simulink model "simplemedusa_model"  (R2020a)
settings: Solver=VariableStepAuto  StartTime=0.0  StopTime=CONSTANTS.T  RelTol=1e-3
model workspace (MAT data in the model file):
  CONSTANTS.MODELPARAMS.mass = 17
  CONSTANTS.MODELPARAMS.I_z = 1
  CONSTANTS.MODELPARAMS.X_dot_u = -20
  CONSTANTS.MODELPARAMS.Y_dot_v = -30
  CONSTANTS.MODELPARAMS.N_dot_r = -8.69
  CONSTANTS.MODELPARAMS.X_u = -0.2
  CONSTANTS.MODELPARAMS.Y_v = -50
  CONSTANTS.MODELPARAMS.N_r = -4.14
  CONSTANTS.MODELPARAMS.X_uu = -25
  CONSTANTS.MODELPARAMS.Y_vv = -0.01
  CONSTANTS.MODELPARAMS.N_rr = -6.23
  CONSTANTS.MODELPARAMS.m_u = 37
  CONSTANTS.MODELPARAMS.m_v = 47
  CONSTANTS.MODELPARAMS.m_r = 9.69
  CONSTANTS.MODELPARAMS.m_uv = -10
  CONSTANTS.MODELPARAMS.fu = 0
  CONSTANTS.MODELPARAMS.fv = 0
  CONSTANTS.MODELPARAMS.fr = 0
  CONSTANTS.MODELPARAMS.Vcx = 0
  CONSTANTS.MODELPARAMS.Vcy = 0
  CONSTANTS.T = 15
  CONSTANTS.xi = [0 0 0 1 0 0]
  CONSTANTS.xf = [15 0 0 1 0 0]
  CONSTANTS.N = 30
  CONSTANTS.obstacles = []
  CONSTANTS.obstacles_circles = []
  CONSTANTS.min_dist_intervehicles = 3
  CONSTANTS.DiffMat = [-2 -0.0666666666667 0 0 0 0 0 0 0 0 0 0 ... (961 elements, 31x31)]
  CONSTANTS.EvalMat = [1 0.361661513462 0.1262127701 0.0423911582752 0.0136635263144 0.00421272023309 0.00123794003929 0.00034530068424 9.10002914127e-05 2.25393402907e-05 5.21509505085e-06 1.11936155556e-06 ... (961 elements, 31x31)]
  CONSTANTS.BigElevMat = [1 0.9 0.809698996656 0.728185674845 0.654631566274 0.588283772395 0.528458304016 0.47453398728 0.425946889606 0.382185222866 0.342784684426 0.30732419983 ... (9331 elements, 301x31)]
  CONSTANTS.numvars = 6
  CONSTANTS.numinputs = 2
  CONSTANTS.Nv = 1
  CONSTANTS.uselogbar = 0
  CONSTANTS.usesigma = 1
  CONSTANTS.statebounds = [-100  -100  -100  -100  -100  -100; 100  100  100  100  100  100]
  CONSTANTS.inputbounds = [-100  -500; 100  500]
  CONSTANTS.costfun_single : function handle (value not decoded)
  CONSTANTS.dynamics : function handle (value not decoded)
  CONSTANTS.init_guess : function handle (value not decoded)
  CONSTANTS.recoverxy : function handle (value not decoded)
  init_vals = [0 0 0 1 0 0]
  tau_r = [43.137679435; -49.2714696293; 18.7459499295; -4.54662431489; 6.658047137; 13.2270237858; 11.3261149802; -5.40954170829; 2.88065093377; -8.94479642329; -0.278054380158; -1.20355590744; 3.44120490313; 2.32411595817; -0.203876719026; 1.93362993926; -0.957580280562; -0.359407602556; 1.46637180945; -1.70192437834; 1.82794903823; -1.09013224286; 0.795656971372; -0.229115148479; 0.177399034781; -0.0352838490099; -0.0922338252967; -0.23784107908; -0.358640517482; -0.316734931346; 0.333994448023]
  tau_u = [19.7607060301; 12.9276910923; 5.53573475394; 4.05635814498; -0.69958092646; 4.06715022134; -3.35509577272; 4.00552304303; -5.80965699996; 11.9065756877; -1.60028180312; 19.6479288494; 1.90021340601; 15.5960881126; 7.73787556532; 8.16534647911; 12.3908641622; 5.37909869708; 12.5613293191; 6.97515929299; 10.8367698131; 8.90302526194; 10.1461113341; 10.1316611384; 10.871270906; 11.7672320885; 13.2342568079; 15.5312905623; 19.2247320659; 25.3375478214; 35.9280012744]
settings Model: Creator=thomas  LastModifiedBy=thomas

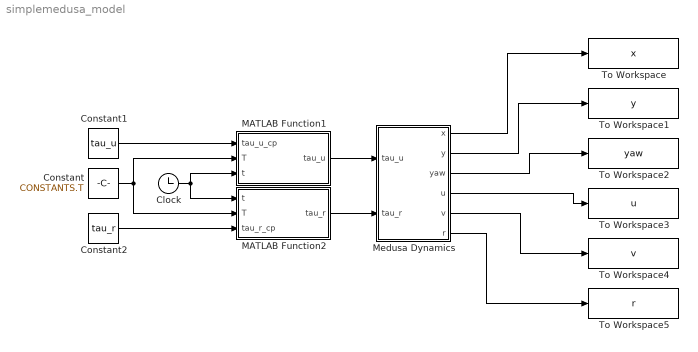
== system simplemedusa_model ==
  Clock : Clock
  Constant : Constant  Value=CONSTANTS.T
  Constant1 : Constant  Value=tau_u
  Constant2 : Constant  Value=tau_r
  MATLAB Function1 : MATLAB Function  TreatAsAtomicUnit=on
  MATLAB Function2 : MATLAB Function  TreatAsAtomicUnit=on
  Medusa Dynamics : Subsystem  mask{x0=init_vals(1), y0=init_vals(2), yaw0=init_vals(3), u0=init_vals(4), v0=init_vals(5), r0=init_vals(6), dist_u=CONSTANTS.MODELPARAMS.fu, dist_v=CONSTANTS.MODELPARAMS.fv, dist_r=CONSTANTS.MODELPARAMS.fr, Vcx=CONSTANTS.MODELPARAMS.Vcx, Vcy=CONSTANTS.MODELPARAMS.Vcy}
      mask prompts: dist_u "Disturbance in u"; dist_v "Disturbance in v"; dist_r "Disturbance in r"; Vcx "Current x"; Vcy "Current y"
  To Workspace : ToWorkspace  VariableName=x  SaveFormat=Structure With Time  SampleTime=-1
  To Workspace1 : ToWorkspace  VariableName=y  SaveFormat=Structure With Time  SampleTime=-1
  To Workspace2 : ToWorkspace  VariableName=yaw  SaveFormat=Structure With Time  SampleTime=-1
  To Workspace3 : ToWorkspace  VariableName=u  SaveFormat=Structure With Time  SampleTime=-1
  To Workspace4 : ToWorkspace  VariableName=v  SaveFormat=Structure With Time  SampleTime=-1
  To Workspace5 : ToWorkspace  VariableName=r  SaveFormat=Structure With Time  SampleTime=-1
  wires:
  MATLAB Function1/1(tau_u) -> Medusa Dynamics/1(tau_u)
  Clock/1 -> MATLAB Function2/1(t), MATLAB Function1/3(t)
  MATLAB Function2/1(tau_r) -> Medusa Dynamics/2(tau_r)
  Constant/1 -> MATLAB Function1/2(T), MATLAB Function2/2(T)
  Constant1/1 -> MATLAB Function1/1(tau_u_cp)
  Constant2/1 -> MATLAB Function2/3(tau_r_cp)
  Medusa Dynamics/1(x) -> To Workspace/1
  Medusa Dynamics/2(y) -> To Workspace1/1
  Medusa Dynamics/3(yaw) -> To Workspace2/1
  Medusa Dynamics/4(u) -> To Workspace3/1
  Medusa Dynamics/5(v) -> To Workspace4/1
  Medusa Dynamics/6(r) -> To Workspace5/1

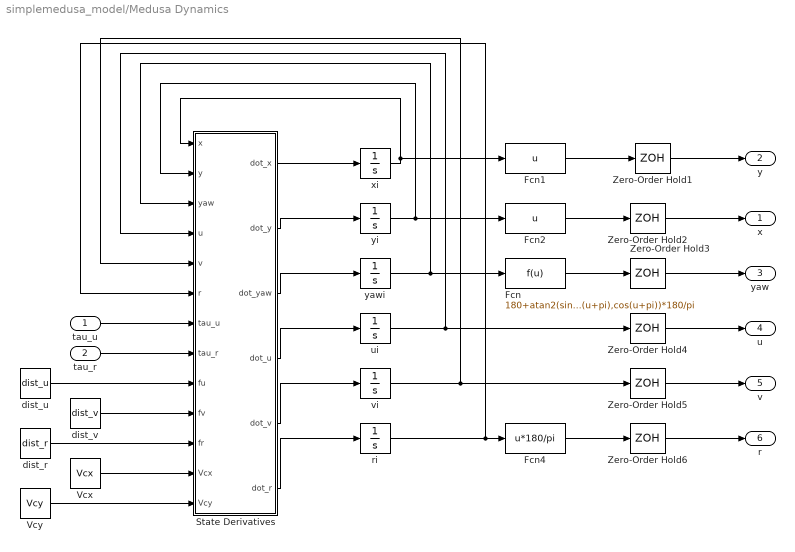
== system simplemedusa_model/Medusa Dynamics ==
  tau_u : Inport
  tau_r : Inport  Port=2
  Fcn : Fcn  Expr=180+atan2(sin(u+pi),cos(u+pi))*180/pi
  Fcn1 : Fcn  Expr=u
  Fcn2 : Fcn  Expr=u
  Fcn4 : Fcn  Expr=u*180/pi
  State Derivatives : MATLAB Function  TreatAsAtomicUnit=on
  Vcx : Constant  Value=Vcx
  Vcy : Constant  Value=Vcy
  Zero-Order Hold{1..6} (6 alike) : ZeroOrderHold  SampleTime=0.2
  dist_r : Constant  Value=dist_r
  dist_u : Constant  Value=dist_u
  dist_v : Constant  Value=dist_v
  ri : Integrator  InitialCondition=r0
  ui : Integrator  InitialCondition=u0
  vi : Integrator  InitialCondition=v0
  xi : Integrator  InitialCondition=y0
  yawi : Integrator  InitialCondition=yaw0
  yi : Integrator  InitialCondition=x0
  x : Outport
  y : Outport  Port=2
  yaw : Outport  Port=3
  u : Outport  Port=4
  v : Outport  Port=5
  r : Outport  Port=6
  wires:
  Fcn4/1 -> Zero-Order Hold6/1
  State Derivatives/1(dot_x) -> xi/1
  State Derivatives/2(dot_y) -> yi/1
  State Derivatives/3(dot_yaw) -> yawi/1
  State Derivatives/4(dot_u) -> ui/1
  State Derivatives/5(dot_v) -> vi/1
  State Derivatives/6(dot_r) -> ri/1
  tau_u/1 -> State Derivatives/7(tau_u)
  yi/1 -> State Derivatives/2(y), Fcn2/1
  xi/1 -> State Derivatives/1(x), Fcn1/1
  yawi/1 -> Fcn/1, State Derivatives/3(yaw)
  ui/1 -> State Derivatives/4(u), Zero-Order Hold4/1
  ri/1 -> Fcn4/1, State Derivatives/6(r)
  vi/1 -> State Derivatives/5(v), Zero-Order Hold5/1
  tau_r/1 -> State Derivatives/8(tau_r)
  dist_u/1 -> State Derivatives/9(fu)
  dist_v/1 -> State Derivatives/10(fv)
  dist_r/1 -> State Derivatives/11(fr)
  Fcn/1 -> Zero-Order Hold3/1
  Vcx/1 -> State Derivatives/12(Vcx)
  Vcy/1 -> State Derivatives/13(Vcy)
  Fcn1/1 -> Zero-Order Hold1/1
  Fcn2/1 -> Zero-Order Hold2/1
  Zero-Order Hold1/1 -> y/1
  Zero-Order Hold2/1 -> x/1
  Zero-Order Hold3/1 -> yaw/1
  Zero-Order Hold4/1 -> u/1
  Zero-Order Hold5/1 -> v/1
  Zero-Order Hold6/1 -> r/1

== matlab function simplemedusa_model/MATLAB Function1 ==
  data: tau_u_cp input; T input; tau_u output; t input
function tau_u = fcn(tau_u_cp, T,t)

coder.extrinsic('BernsteinEval') 
tau_u=0;
tau_u = BernsteinEval(tau_u_cp, T, t);

end

== matlab function simplemedusa_model/MATLAB Function2 ==
  data: t input; T input; tau_r_cp input; tau_r output
function tau_r = fcn(t,T, tau_r_cp)

coder.extrinsic('BernsteinEval') 
tau_r=0;
tau_r = BernsteinEval(tau_r_cp, T, t);

end

== matlab function simplemedusa_model/Medusa Dynamics/State Derivatives ==
  data: x input; y input; yaw input; u input; v input; r input; tau_u input; dot_x output; tau_r input; dot_y output; dot_yaw output; dot_u output; dot_v output; dot_r output; fu input; fv input; fr input; Vcx input; Vcy input
function [dot_x,dot_y,dot_yaw,dot_u,dot_v,dot_r] = fcn(x,y,yaw,u,v,r,tau_u,tau_r,fu,fv,fr, Vcx, Vcy)
%state = [x, y, yaw, u, v, r]

% %%%%%% Coefficients
% mass = 17.0;
% I_z = 4.14;
% X_dot_u = -20;
% Y_dot_v = -1.3175;
% N_dot_r =  -8.69;
% X_u = -0.2;
% Y_v = -55.117;
% N_r = -4.14;
% X_uu = -25; 
% Y_vv = -101.2776;
% N_rr = -6.23;

%%%%%% Coefficients
mass = 17.0;
I_z = 1;
X_dot_u = -20;
Y_dot_v = -30;%-1.3175;
N_dot_r = -8.69;% -0.5;
X_u = -0.2;
Y_v = -50;
N_r = -4.14; %-0.1
X_uu = -25; 
Y_vv = -0.01;%-101.2776;
N_rr = -6.23; %-21

%%%%%% masses
m_u = mass - X_dot_u;
m_v = mass - Y_dot_v;
m_r = I_z - N_dot_r;
m_uv = m_u - m_v;

%%%%%%%%% drag

d_u = -X_u - X_uu*abs(u);
d_v = -Y_v - Y_vv*abs(v);
d_r = -N_r - N_rr*abs(r);

%%%%%%%%% Dynamics

dot_u = 1/m_u*(tau_u + m_v*v*r - d_u*u+fu);
dot_v = 1/m_v*(-m_u*u*r - d_v*v+fv);
dot_r = 1/m_r*(tau_r + m_uv*u*v - d_r*r+fr);

dot_x = u*cos(yaw) - v*sin(yaw) + Vcx;
dot_y = u*sin(yaw) + v*cos(yaw) + Vcy;
dot_yaw = r;
